simulink model "exercise3"  (R2017a)
settings: Solver=VariableStepAuto  StartTime=0.0  StopTime=10.0  RelTol=1e-3
values from neighbouring files (symbols this model uses):
  g = 9.8    [pendel3.mat]    (also in stuff.m = 9.82)
  l = 0.7    [pendel3.mat]    (also in stuff.m)
  M = 0.5    [pendel3.mat]    (also in stuff.m)
settings Model: Creator=viktor  LastModifiedBy=viktor

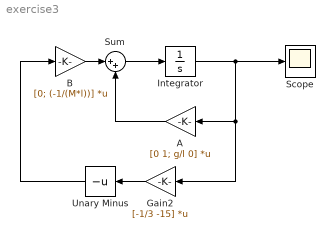
== system exercise3 ==
  A : Gain  Gain=[0 1; g/l 0]  Multiplication=Matrix(K*u)
  B : Gain  Gain=[0; (-1/(M*l))]  Multiplication=Matrix(K*u)
  Gain2 : Gain  Gain=[-1/3 -15]  Multiplication=Matrix(K*u)
  Integrator : Integrator  InitialCondition=[30; 0]
  Scope : Scope
  Sum : Sum  Inputs=|++
  Unary Minus : UnaryMinus
  wires:
  B/1 -> Sum/1
  Gain2/1 -> Unary Minus/1
  A/1 -> Sum/2
  Sum/1 -> Integrator/1
  Integrator/1 -> Scope/1, Gain2/1, A/1
  Unary Minus/1 -> B/1
